simulink model "LQR_Control_Model_png"  (R2018b)
settings: Solver=ode1  StartTime=0.0  StopTime=10  FixedStep=0.001  MaxStep=0.001  RelTol=1e-3
InitFcn:
  | close all;
  | clc;
  | clear;
StopFcn:
  | position = system_output(:,1);
  | speed = system_output(:,2);
  | angle = system_output(:,3);
  | angular_velocity = system_output(:,4);
  | t = [1:length(position)];
  | 
  | figure;plot(t,position);
  | title('Position');
  | 
  | figure;plot(t,speed);
  | title('Speed');
  | 
  | figure;plot(t,angle);
  | title('Angle');
  | 
  | figure;plot(t,angular_velocity);
  | title('Angle Velocity');
  | 
  | 
  | u_law = control_output(:,1);
  | u_NN = control_output(:,2);
  | u_LQR = control_output(:,3);
  | t = [1:length(u_law)];
  | 
  | figure;plot(t,u_law);
  | title('u law');
  | 
  | figure;plot(t,u_NN);
  | title('u NN');
  | 
  | figure;plot(t,u_LQR);
  | title('u LQR');
undefined symbols (not defined in the file or in its folder): sigbuilder_block
settings Model: Creator=Lenovo  LastModifiedBy=Richard
settings DataIOCC: LimitDataPoints=on  SaveFormat=Array
settings OptimizationCC: BlockReduction=off  BooleanDataType=off  LifeSpan=inf
settings DebuggingCC: SaveWithParameterizedLinksMsg=none  UnderspecifiedInitializationDetection=Classic  MergeDetectMultiDrivingBlocksExec=none  SignalResolutionControl=TryResolveAllWithWarning  SFUnexpectedBacktrackingDiag=warning  SFNoUnconditionalDefaultTransitionDiag=warning  SFExecutionAtInitializationDiag=none
settings HardwareCC: ProdBitPerPointer=32  ProdBitPerSizeT=32  ProdBitPerPtrDiffT=32  ProdLargestAtomicFloat=None  ProdIntDivRoundTo=Undefined  ProdEndianess=Unspecified  ProdWordSize=32  ProdHWDeviceType=32-bit Generic  TargetUnknown=on
settings ModelReferenceCC: PropagateSignalLabelsOutOfModel=off
settings SFSimCC: SimUseLocalCustomCode=off
settings RTWCC: RTWUseLocalCustomCode=off
settings CodeAppCC: StateflowObjectComments=on
settings GRTTargetCC: TargetLangStandard=C89/C90 (ANSI)  GeneratePreprocessorConditionals=Disable all
settings ConfigComp: CovMetricSettings=dw  CovHtmlReporting=on  CovSaveCumulativeToWorkspaceVar=on  CovSaveSingleToWorkspaceVar=on  CovExternalEMLEnable=off  CovSFcnEnable=off

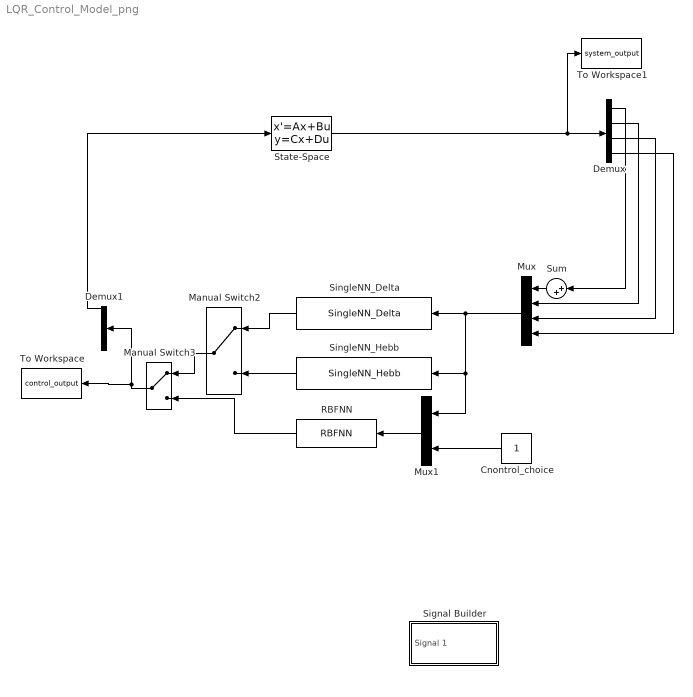
== system LQR_Control_Model_png ==
  Cnontrol_choice : Constant
  Demux : Demux
  Demux1 : Demux  Outputs=5
  Manual Switch2 : ManualSwitch
  Manual Switch3 : ManualSwitch
  Mux : Mux
  Mux1 : Mux  Inputs=2
  RBFNN : S-Function  FunctionName=RBFNN  SFunctionDeploymentMode=off  EnableBusSupport=off
  Signal Builder : Subsystem  Tag=STV Subsys  LoadFcn=sigbuilder_block('load');  StartFcn=sigbuilder_block('start');  StopFcn=sigbuilder_block('stop');  ClipboardFcn=sigbuilder_block('clipboard');  mask(Sigbuilder block){tuvar=[0:10]}
      mask help: Simulink:masks:SigbuilderBlock_MD
      mask init:
      | if ~strcmp(get_param(bdroot(gcbh),'SimulationStatus'),'stopped') tuvar = sigbuilder_block('maskInit'); end
      settings: CopyFcn=sigbuilder_block('copy');  DeleteFcn=sigbuilder_block('delete');  ModelCloseFcn=sigbuilder_block('modelClose');  PreSaveFcn=sigbuilder_block('preSave');  PauseFcn=sigbuilder_block('pause');  ContinueFcn=sigbuilder_block('continue');  NameChangeFcn=sigbuilder_block('namechange');  OpenFcn=sigbuilder_block('open',[437.6 199.2 550.4 400 ]);  CloseFcn=sigbuilder_block('close');
      mask Display: plot(0, 0, 100, 100,[2, 2, 32, 32, 2], [68, 8, 8, 68, 68],[32, 2], [38, 38], [32, 19, 2],[53, 60, 44], [32, 17, 17, 2],[16, 16, 31, 31]);txt = getActiveGroup(gcbh);text(2, 100, txt,'verticalAlignment', 'top');
  SingleNN_Delta : S-Function  FunctionName=SingleNN_Delta  SFunctionDeploymentMode=off  EnableBusSupport=off
  SingleNN_Hebb : S-Function  FunctionName=SingleNN_Hebb  SFunctionDeploymentMode=off  EnableBusSupport=off
  State-Space : StateSpace  A=[0 1 0 0;0 -0.1164 1.2373 0;0 0 0 1;0 -0.7164 67.9221 0]  B=[0;1.4554;0;8.9546]  C=[1 0 0 0;0 1 0 0;0 0 1 0;0 0 0 1]  D=[0;0;0;0]  InitialCondition=[1;1;1;1]
  Sum : Sum  Inputs=|++
  To Workspace : ToWorkspace  VariableName=control_output  SampleTime=-1
  To Workspace1 : ToWorkspace  VariableName=system_output  SampleTime=-1
  wires:
  Demux/1 -> Sum/1
  Demux/2 -> Mux/2
  Demux/4 -> Mux/4
  Demux/3 -> Mux/3
  Demux1/1 -> State-Space/1
  SingleNN_Delta/1 -> Manual Switch2/1
  SingleNN_Hebb/1 -> Manual Switch2/2
  Mux/1 -> Mux1/1, SingleNN_Hebb/1, SingleNN_Delta/1
  Manual Switch2/1 -> Manual Switch3/1
  RBFNN/1 -> Manual Switch3/2
  Cnontrol_choice/1 -> Mux1/2
  Mux1/1 -> RBFNN/1
  Sum/1 -> Mux/1
  Manual Switch3/1 -> Demux1/1, To Workspace/1
  State-Space/1 -> To Workspace1/1, Demux/1

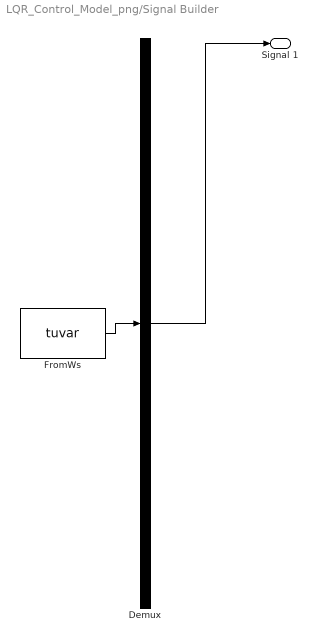
== system LQR_Control_Model_png/Signal Builder ==
  Demux : Demux  Tag=STV Demux  Outputs=1
  FromWs : FromWorkspace  Tag=STV FromWs  VariableName=tuvar  SampleTime=0
      SigBuilderData=|
      | common.afterFinalStr = 'Extrapolate'
      | common.sampleTime = 0
      | dataSet.timeRange = [0 10]
      | dataSet.name = 'Group 1'
      | sbobj.Groups.Name = 'Group 1'
      | sbobj.Groups.Signals.Name = 'Signal 1'
      | sbobj.Groups.Signals.XData = [0 4 4 10]
      | sbobj.Groups.Signals.YData = [0 0 1 1]
  Signal 1 : Outport  Tag=STV Outport
  wires:
  Demux/1 -> Signal 1/1
  FromWs/1 -> Demux/1
